simulink model "natnetTest"  (R2022b)
settings: Solver=FixedStepAuto  StartTime=0.0  StopTime=5  RelTol=1e-3
values from neighbouring files (symbols this model uses):
  natnetclient = natnet    [NatNetPollingErrorInCircle.m]    (also in intializeMotiveObject.m = []; natnetTestSetup.m = intializeMotiveObject())
  sampleTime = 0.01    [natnetTestSetup.m]
undefined symbols (not defined in the file or in its folder): motiveGetFrameData
libraries: sldrtlib x1, slrealtimeiplib x1
settings Model: Creator=hu650776  LastModifiedBy=hu650776
settings SolverCC: ConcurrentTasks=on  AlgebraicLoopSolver=TrustRegion  DecoupledContinuousIntegration=on  MinimalZcImpactIntegration=on
settings DebuggingCC: UnconnectedInputMsg=warning  UnconnectedOutputMsg=warning  UnconnectedLineMsg=warning  SFMachineParentedDataDiag=warning  ArithmeticOperatorsInVariantConditions=warning
settings HardwareCC: ProdBitPerLong=64  ProdHWDeviceType=Intel->x86-64 (Linux 64)
settings ModelReferenceCC: EnableRefExpFcnMdlSchedulingChecks=on
settings SFSimCC: SimUseLocalCustomCode=off  CustomCodeUndefinedFunction=UseInterfaceOnly
settings RTWCC: Description=Simulink Desktop Real-Time  SystemTargetFile=sldrt.tlc  TemplateMakefile=sldrt.tmf  RTWUseLocalCustomCode=off  RTWCompilerOptimization=on  DLArmComputeVersion=19.05
settings CodeAppCC: MaxIdLength=95
settings SimulinkDesktopRealTimeCC: TargetLibSuffix=_sldrt.a  TargetPreCompLibLocation=C:\Users\hu650776\MATLAB\toolbox\sldrt\lib\win64

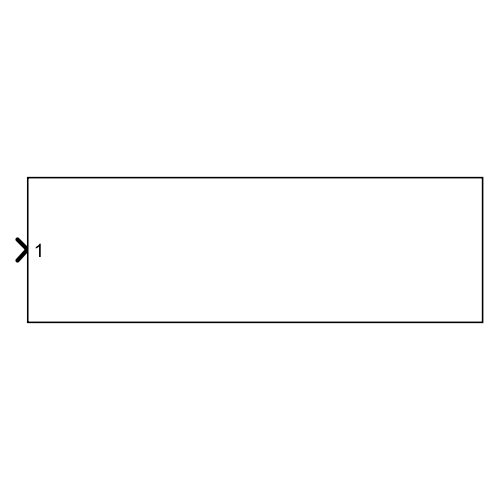
[thumbnail: Simulink's stored preview of the top-level diagram]
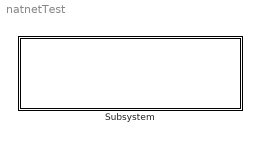
== system natnetTest ==
  Subsystem : Subsystem

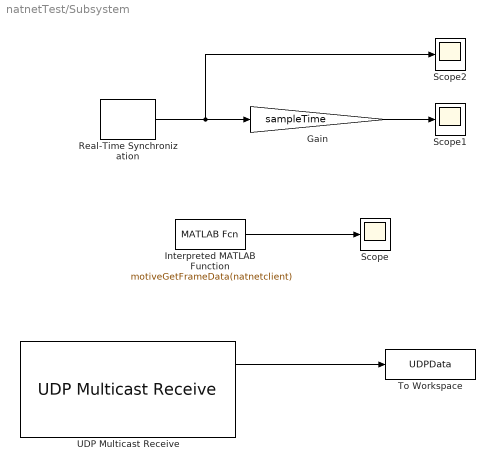
== system natnetTest/Subsystem ==
  Gain : Gain  Gain=sampleTime
  Interpreted MATLAB Function : MATLABFcn  MATLABFcn=motiveGetFrameData(natnetclient)  OutputDimensions=1  Output1D=off
  Real-Time Synchronization : sldrtlib/Real-Time Synchronization  SampleTime=sampleTime  MaxMissedTicks=Inf  ShowMissedTicks=on  YieldWhenWaiting=off
  Scope : Scope
  Scope1 : Scope
  Scope2 : Scope
  To Workspace : ToWorkspace  VariableName=UDPData  SaveFormat=Timeseries  SampleTime=-1
  UDP Multicast Receive : slrealtimeiplib/UDP Multicast Receive  bindAddress=0.0.0.0  localPort=1511  rcvWidth=-1  multicastAddress={'239.255.42.99'}  multicastInterface={'127.0.0.1'}  sampleTime=sampleTime
  wires:
  Real-Time Synchronization/1 -> Scope2/1, Gain/1
  Gain/1 -> Scope1/1
  Interpreted MATLAB Function/1 -> Scope/1
  UDP Multicast Receive/1 -> To Workspace/1
